simulink model "self_triggered_mpc_simulation"  (R2023a)
settings: Solver=VariableStepAuto  StartTime=0.0  StopTime=param.Tsim  RelTol=1e-3
values from neighbouring files (symbols this model uses):
  param = struct    [autometica_mpc.m]    (also in cost_cal.m = param_setup(); main.m = param_setup(); para.m; param.mat = )
settings Model: Creator=김준수  LastModifiedBy=김준수

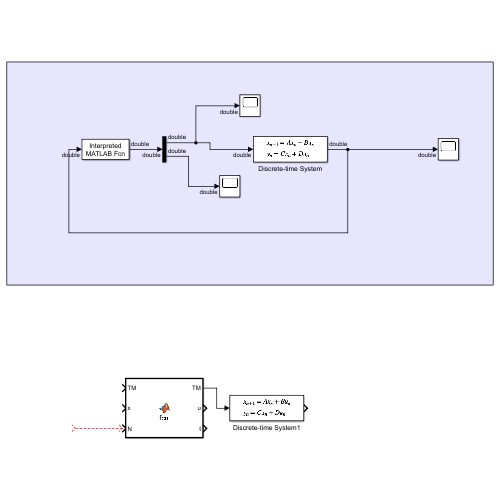
[thumbnail: Simulink's stored preview of the top-level diagram]
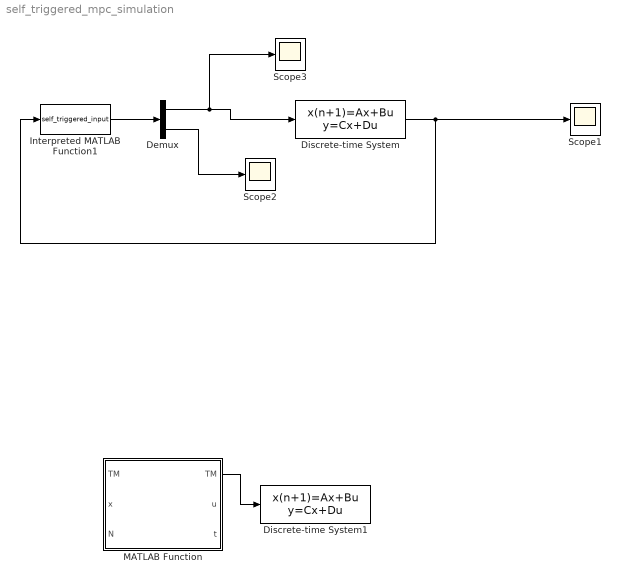
== system self_triggered_mpc_simulation ==
  Demux : Demux  Outputs=2
  Discrete-time System : DiscreteStateSpace  A=param.A  B=param.B  C=eye(param.nx)  D=zeros(param.nx,1)  InitialCondition=param.x0
  Discrete-time System1 : DiscreteStateSpace  A=param.A  B=param.B  C=eye(param.nx)  D=zeros(param.nx,1)  InitialCondition=param.x0
  Interpreted MATLAB Function1 : MATLABFcn  MATLABFcn=self_triggered_input  OutputDimensions=param.nu+1  Output1D=off
  MATLAB Function : MATLAB Function  TreatAsAtomicUnit=on
  Scope1 : Scope
  Scope2 : Scope
  Scope3 : Scope
  wires:
  Discrete-time System/1 -> Scope1/1, Interpreted MATLAB Function1/1
  Interpreted MATLAB Function1/1 -> Demux/1
  Demux/1 -> Scope3/1, Discrete-time System/1
  Demux/2 -> Scope2/1
  MATLAB Function/1(TM) -> Discrete-time System1/1
  ? -> ?

== matlab function self_triggered_mpc_simulation/MATLAB Function ==
  data: TM output; TM input; x input; N input; u output; t output
function [TM, u, t] = fcn(TM, x, N)

%==========================================================================
%parameter setting
param = param_setup
coder.extrinsic("optimconstr", "optimproblem", "optimvar");
prob = optimproblem;
x0 = optimvar('x0', param.nx);
x = optimvar('x', param.nx,N);
u0 = optimvar('x', param.nu);
u = optimvar('u',param.nu, N-1);

cost_function =x0'*param.Q*x0+u0*param.R*u0;


y= 0;
